simulink model "fuel1"  (R2021a)
settings: Solver=VariableStepAuto  StartTime=0.0  StopTime=10.0  RelTol=1e-3
libraries: spsFuelCellStackLib x1, spsSeriesRLCBranchLib x1, spsVoltageMeasurementLib x1, spspowerguiLib x1
settings Model: Creator=LENOVO  LastModifiedBy=LENOVO

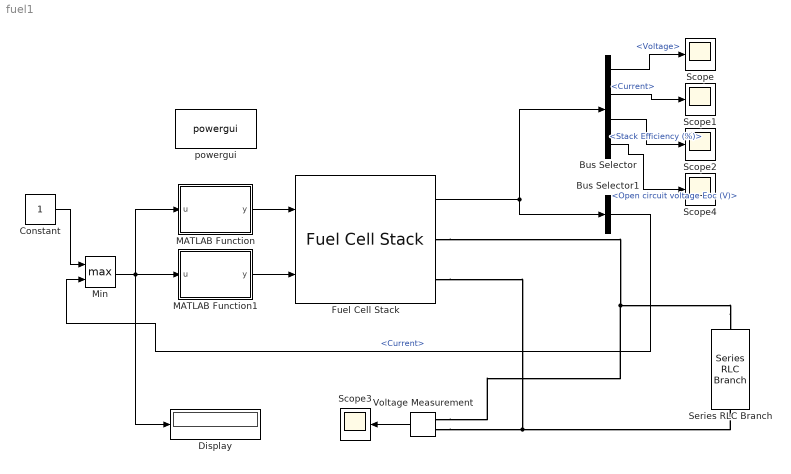
== system fuel1 ==
  Bus Selector : BusSelector  OutputSignals=Voltage,Current,Stack Efficiency (%),Open circuit voltage Eoc (V)
  Bus Selector1 : BusSelector  OutputSignals=Current
  Constant : Constant
  Display : Display
  Fuel Cell Stack : spsFuelCellStackLib/Fuel Cell Stack  PresetModel=No (User-Defined)  FcType=0  Detailed=Detailed  Eoc=[42,35]  NomVI=[52,24.23]  EndVI=[100,20]  Nc=20  n=46  TOp=55  AirFr=2400  SuppPress=[1.5,1]  Comp=[99.95,21,1]  SignX=off  SignY=off  FlowRateH2=on  FlowRateAir=on  SystemTemp=off  SystemPH2=off  SystemPAir=off  FCDyn=off  FC_tau=1  Peak_O2=80  V_Under=10
      settings: SourceProductBaseCode=PS
  MATLAB Function : MATLAB Function  TreatAsAtomicUnit=on
  MATLAB Function1 : MATLAB Function  TreatAsAtomicUnit=on
  Min : MinMax  Function=max  Inputs=2
  Scope{,1..4} (5 alike) : Scope
  Series RLC Branch : spsSeriesRLCBranchLib/Series RLC Branch  LConnTagsString=__new0  RConnTagsString=__new0  BranchType=R  Resistance=10  Inductance=1e-3  SetiL0=off  InitialCurrent=0  Capacitance=1e-6  Setx0=off  InitialVoltage=0  Measurements=None
  Voltage Measurement : spsVoltageMeasurementLib/Voltage Measurement  PhasorSimulation=off  OutputType=Complex  PSBequivalent=0
  powergui : spspowerguiLib/powergui  Priority=1  SimulationMode=Continuous  SampleTime=50e-6  frequency=60  Iterations=50  frequencyindice=0  Pbase=100e6  ErrMax=1e-4  UnitsV=kV  UnitsW=MW  buscounter=0  FunctionMessages=off  echomessages=off  EnableUseOfTLC=off  CurrentSourceSwitches=off  DisableSnubberDevices=off  DisableRonSwitches=off  DisableVfSwitches=off  DisplayEquations=off  AutomaticDiscreteSolvers=off  SolverType=Tustin/Backward Euler (TBE)  Interpol=off  ExternalGateDelay=off  methode=off  Ts=100  x0status=blocks  SPID=on  SwTol=0  HookPort=off  NonlinearTolerance=1e-4  nMaxIteration=100  ContinueOnMaxIteration=off  RestoreLinks=warning  ResistiveCurrentMeasurement=off  Frange=[0:2:500]  Ylog=off  Xlog=on  ShowGrid=off  save=off  variable=ZData  structure=0  ZoomFFT=off  StartTime=0.0  cycles=1  DisplayStyle=1  fundamental=60  FreqAxis=off  MaxFrequency=1000  frequencyindicesteady=1  RmsSteady=1  display=off
  wires:
  Constant/1 -> Min/1
  Bus Selector1/1 -> Min/2  "<Current>"
  Bus Selector/3 -> Scope2/1  "<Stack Efficiency (%)>"
  Bus Selector/2 -> Scope1/1  "<Current>"
  MATLAB Function1/1(y) -> Fuel Cell Stack/2
  Bus Selector/1 -> Scope/1  "<Voltage>"
  Voltage Measurement/1 -> Scope3/1
  MATLAB Function/1(y) -> Fuel Cell Stack/1
  Fuel Cell Stack/1 -> Bus Selector/1, Bus Selector1/1
  Bus Selector/4 -> Scope4/1  "<Open circuit voltage Eoc (V)>"
  Min/1 -> MATLAB Function1/1(u), MATLAB Function/1(u), Display/1
  connections:
  Fuel Cell Stack/RConn2 -- Series RLC Branch/RConn1 -- Voltage Measurement/LConn2
  Series RLC Branch/LConn1 -- Voltage Measurement/LConn1 -- Fuel Cell Stack/RConn1

== matlab function fuel1/MATLAB Function ==
  data: u input; y output
function y = fcn(u)
60000*8.3145*(273+95)*400*u(1)/(2*96485*(3*101325)*0.919*0.995)
y = u;

== matlab function fuel1/MATLAB Function1 ==
  data: u input; y output
function y = fcn(u)
60000*8.3145*(273+95)*400*u(1)/(4*96485*(3*101325)*0.5057*0.21)

y = u;
